simulink model "sl_quadrotor_vs"  (R2018a)
settings: Solver=ode45  StartTime=0.0  StopTime=10  RelTol=1e-3  EnableMultiTasking=on
InitFcn:
  | fprintf('----- creating workspace variables: camera, quad, P, pstar\n');
  | % create a spherical camera
  | camera = SphericalCamera('name', 'quad-vs');
  | 
  | % create a grid of points on the ground
  | P = mkgrid(2, 4);
  | 
  | % set the desired view of these points, defines the final pose
  | % of the quad
  | pstar = camera.project(P, 'pose', SE3(0, 0, -5)*SE3.Rz(pi/2));
  | 
  | % load a dynamic model of the quadrotor
  | mdl_quadrotor
undefined symbols (not defined in the file or in its folder): rpy2tr, transl
libraries: roblocks x8
settings Model: Creator=corkep  LastModifiedBy=corkep
settings OptimizationCC: ExpressionDepthLimit=2147483647  LifeSpan=inf
settings DebuggingCC: UnderspecifiedInitializationDetection=Classic  MergeDetectMultiDrivingBlocksExec=none  SolverPrmCheckMsg=warning  AllowSymbolicDim=off  StateNameClashWarn=warning  SFUnexpectedBacktrackingDiag=warning  SFNoUnconditionalDefaultTransitionDiag=warning  SFExecutionAtInitializationDiag=none
settings HardwareCC: ProdBitPerPointer=32  ProdBitPerSizeT=32  ProdBitPerPtrDiffT=32  ProdLargestAtomicFloat=None  ProdIntDivRoundTo=Undefined  ProdEndianess=Unspecified  ProdWordSize=32  ProdHWDeviceType=32-bit Generic
settings ModelReferenceCC: PropagateSignalLabelsOutOfModel=off
settings CodeAppCC: StateflowObjectComments=on
settings GRTTargetCC: TargetLangStandard=C89/C90 (ANSI)  GeneratePreprocessorConditionals=Disable all  CombineOutputUpdateFcns=off  GRTInterface=on
settings ConfigComp: CovMetricSettings=dw  CovHtmlReporting=on  CovSaveCumulativeToWorkspaceVar=on  CovSaveSingleToWorkspaceVar=on  CovExternalEMLEnable=off  CovSFcnEnable=off

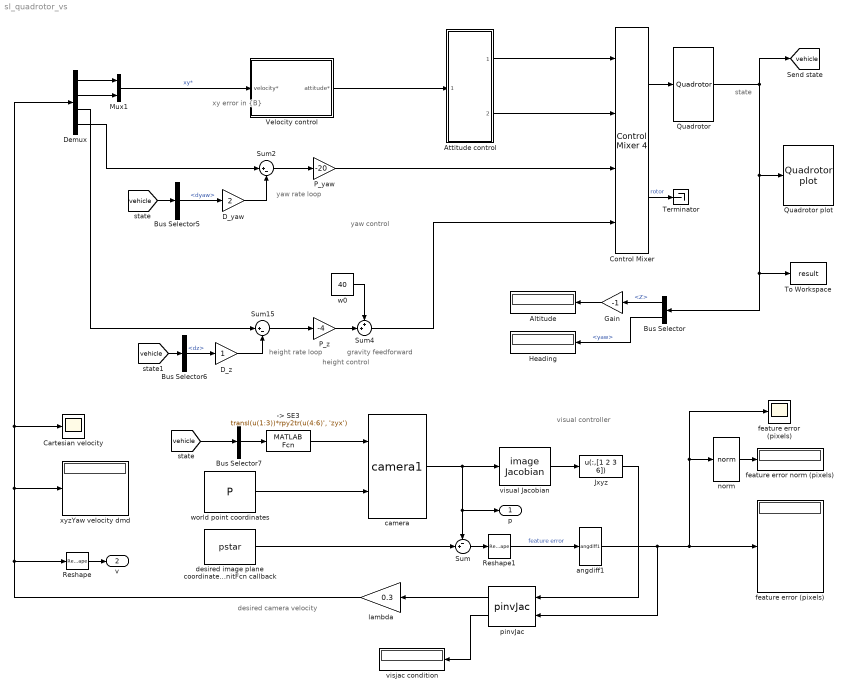
== system sl_quadrotor_vs ==
  note: visual controller
  note: state
  note: xy error
      | in {B}
  note: yaw rate
      | loop
  note: yaw control
  note: height rate
      | loop
  note: gravity feedforward
  note: height control
  note: desired camera velocity
  -> SE3 : MATLABFcn  MATLABFcn=transl(u(1:3))*rpy2tr(u(4:6)', 'zyx')  OutputDimensions=[4 4]  Output1D=off
  Altitude : Display
  Attitude control : Subsystem  mask{P=100, D=1}
      mask prompts: P "Proportional gain"; D "Derivative gain"
  Bus Selector : BusSelector  OutputSignals=Z,yaw
  Bus Selector5 : BusSelector  OutputSignals=dyaw
  Bus Selector6 : BusSelector  OutputSignals=dz
  Bus Selector7 : BusSelector  OutputSignals=X,Y,Z,roll,pitch,yaw  OutputAsBus=on
  Cartesian velocity : Scope
  Control Mixer : roblocks/Vehicles/Control Mixer 4  quad=quadrotor  maxrot=1000  minrot=5
  D_yaw : Gain  Gain=2
  D_z : Gain
  Demux : Demux
  Gain : Gain  Gain=-1
  Heading : Display
  Jxyz : MATLABFcn  MATLABFcn=u(:,[1 2 3 6])  Output1D=off
  Mux1 : Mux  Inputs=2
  P_yaw : Gain  Gain=-20
  P_z : Gain  Gain=-4
  Quadrotor : roblocks/Vehicles/Quadrotor  quad=quadrotor  x0=[0 0 -0.2]  groundflag=on
  Quadrotor plot : roblocks/Vehicles/Quadrotor plot  quad=quadrotor  xydim=2  zdim=10
  Reshape : Reshape  OutputDimensions=6
  Reshape1 : Reshape  OutputDimensions=6
  Sum : Sum  Inputs=-+|  SaturateOnIntegerOverflow=on  InputSameDT=on  OutDataTypeStr=Inherit: Same as first input
  Sum15 : Sum  Inputs=|+-
  Sum2 : Sum  Inputs=|+-
  Sum4 : Sum  Inputs=++|
  Terminator : Terminator
  To Workspace : ToWorkspace  VariableName=result  SampleTime=-1
  Velocity control : Subsystem  mask{P=0.1, D=2}
      mask prompts: P "Proportional gain"; D "Derivative gain"
  angdiff1 : roblocks/Toolbox/angdiff1
  camera : roblocks/Vision/camera1  cam=camera
  desired image plane coordinates (pixels) **set in model InitFcn callback : Constant  Value=pstar  VectorParams1D=off
  feature error norm (pixels) : Display
  feature error (pixels) : Display
      settings: Format=bank
  "feature error (pixels) " : Scope
  lambda : Gain  Gain=0.3  SaturateOnIntegerOverflow=on  OutDataTypeStr=Inherit: Same as input  ParamDataTypeStr=Inherit: Same as input
  norm : roblocks/Toolbox/norm  SystemSampleTime=-1
  pinvJac : roblocks/Toolbox/pinvJac
  visjac condition : Display
  visual Jacobian : roblocks/Vision/image Jacobian  cam=camera  z=3
  w0 : Constant  Value=40  SampleTime=0
  world point coordinates : Constant  Value=P  VectorParams1D=off
  xyzYaw velocity dmd : Display
      settings: Format=bank
  p : Outport
  v : Outport  Port=2
  tag scope: vehicle=global
  wires:
  Velocity control/1(attitude*) -> Attitude control/1(attitude*)
  Mux1/1 -> Velocity control/1(velocity*)  "xy*"
  Attitude control/1(roll torque*) -> Control Mixer/1
  Attitude control/2(pitch torque*) -> Control Mixer/2
  Control Mixer/1 -> Quadrotor/1
  Sum4/1 -> Control Mixer/4
  Demux/1 -> Mux1/1
  Demux/2 -> Mux1/2
  Demux/4 -> Sum2/1
  D_yaw/1 -> Sum2/2
  Bus Selector5/1 -> D_yaw/1  "<dyaw>"
  Sum2/1 -> P_yaw/1
  [vehicle] -> Bus Selector5/1
  [vehicle] -> Bus Selector6/1
  D_z/1 -> Sum15/2
  Bus Selector6/1 -> D_z/1  "<dz>"
  P_z/1 -> Sum4/2
  Sum15/1 -> P_z/1
  w0/1 -> Sum4/1
  [vehicle] -> Bus Selector7/1
  Sum/1 -> Reshape1/1
  desired image plane coordinates (pixels) **set in model InitFcn callback/1 -> Sum/2
  Reshape1/1 -> angdiff1/1  "feature error"
  pinvJac/2 -> visjac condition/1
  pinvJac/1 -> lambda/1
  Bus Selector7/1 -> -> SE3/1
  visual Jacobian/1 -> Jxyz/1
  Reshape/1 -> v/1
  camera/1 -> visual Jacobian/1, Sum/1, p/1
  world point coordinates/1 -> camera/2
  norm/1 -> feature error norm (pixels)/1
  Jxyz/1 -> pinvJac/1
  -> SE3/1 -> camera/1
  lambda/1 -> Reshape/1, Demux/1, Cartesian velocity/1, xyzYaw velocity dmd/1
  P_yaw/1 -> Control Mixer/3
  Quadrotor/1 -> Bus Selector/1, To Workspace/1, Quadrotor plot/1, [vehicle]
  Control Mixer/2 -> Terminator/1  "rotor"
  Demux/3 -> Sum15/1
  angdiff1/1 -> feature error (pixels)/1, "feature error (pixels) "/1, norm/1, pinvJac/2
  Bus Selector/1 -> Gain/1  "<Z>"
  Bus Selector/2 -> Heading/1  "<yaw>"
  Gain/1 -> Altitude/1

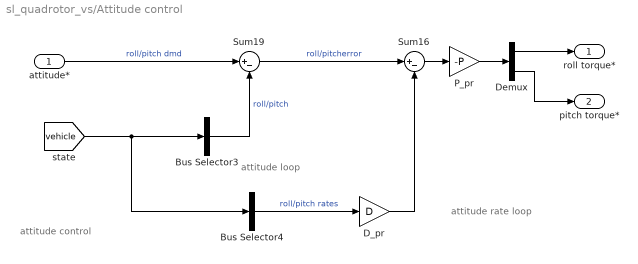
== system sl_quadrotor_vs/Attitude control ==
  note: attitude control
  note: attitude rate loop
  note: attitude loop
  attitude* : Inport
  Bus Selector3 : BusSelector  OutputSignals=roll,pitch  OutputAsBus=on
  Bus Selector4 : BusSelector  OutputSignals=droll,dpitch  OutputAsBus=on
  D_pr : Gain  Gain=D
  Demux : Demux  Outputs=2
  P_pr : Gain  Gain=-P
  Sum16 : Sum  Inputs=|+-
  Sum19 : Sum  Inputs=|+-
  roll torque* : Outport
  pitch torque* : Outport  Port=2
  wires:
  [vehicle] -> Bus Selector4/1, Bus Selector3/1
  attitude*/1 -> Sum19/1  "roll/pitch dmd"
  Bus Selector3/1 -> Sum19/2  "roll/pitch"
  Bus Selector4/1 -> D_pr/1  "roll/pitch rates"
  Sum19/1 -> Sum16/1  "roll/pitcherror"
  Sum16/1 -> P_pr/1
  P_pr/1 -> Demux/1
  D_pr/1 -> Sum16/2
  Demux/2 -> pitch torque*/1
  Demux/1 -> roll torque*/1

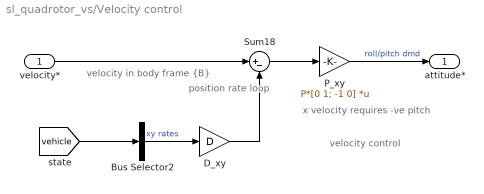
== system sl_quadrotor_vs/Velocity control ==
  note: x velocity requires -ve pitch
  note: velocity in body frame {B}
  note: velocity control
  note: position rate
      | loop
  velocity* : Inport
  Bus Selector2 : BusSelector  OutputSignals=dx,dy  OutputAsBus=on
  D_xy : Gain  Gain=D
  P_xy : Gain  Gain=P*[0 1; -1 0]  Multiplication=Matrix(K*u)
  Sum18 : Sum  Inputs=|+-
  attitude* : Outport
  wires:
  Bus Selector2/1 -> D_xy/1  "xy rates"
  D_xy/1 -> Sum18/2
  Sum18/1 -> P_xy/1
  velocity*/1 -> Sum18/1
  [vehicle] -> Bus Selector2/1
  P_xy/1 -> attitude*/1  "roll/pitch dmd"
